simulink model "BEVModel"  (R2021a)
settings: Solver=ode4  StartTime=0  StopTime=tEnd  FixedStep=dt  RelTol=1e-3
values from neighbouring files (symbols this model uses):
  accessoryLoad = 600    [main.m]
  Af = 1.00    (= 1)    [main.m]
  batteryCapacity = 50    [main.m]
  batteryResistance = 0.0461    [main.m]
  C = 400    [main.m]
  Cd = 0.576    [main.m]
  Crr = 0.01    [main.m]
  cycleNum = 2    [main.m]
  EffTableEff = [.75 .85 .89 .95 .96 .97 .98 .99 .99]    [main.m]
  EffTableSpeed = [0 5 10 15 25 35 45 55 65]    [main.m]
  g = 9.81    [main.m]
  GRd = 9.843    [main.m]
  k_J2gal = 1/3600000/32.3    (= 8.59993120055e-09)    [main.m]
  k_kWh2J = 3.6*10^6    (= 3600000)    [main.m]
  k_m2mi = 0.000621371    [main.m]
  k_rps2rpm = 60/(2*pi)    (= 9.54929658551)    [main.m]
  k_s2h = 1/3600    (= 0.000277777777778)    [main.m]
  k_W2kW = 1/1000    (= 0.001)    [main.m]
  kc = 0.513    [main.m]
  Kd = 0    [main.m]
  Ki = 0.1    [main.m]
  ki = 0.0773    [main.m]
  Kp = 200    [main.m]
  kw = 0.0000064    (= 6.4e-06)    [main.m]
  m = 1965    [main.m]
  motorMaxPower = 310000    [main.m]
  motorMaxSpeed = 18000    [main.m]
  motorMaxTorque = 600    [main.m]
  openCircuitVoltage = 420    [main.m]
  pBrakeMax = 4*TbrakeMax / (mu_k*pi()* cylinderBore^2 *meanPadRadius*numPads)    [main.m]
  r = 0.290    (= 0.29)    [main.m]
  rho = 1.20    (= 1.2)    [main.m]
  SOCi = 90    [main.m]
  theta = 0    [main.m]
  v0 = 0    [main.m]
  x0 = 0    [main.m]
libraries: autolibshared x6, fl_lib x5, nesl_utility x5, sdl_lib x1
settings Model: Creator=Chris  LastModifiedBy=jordan
settings SolverCC: AlgebraicLoopSolver=TrustRegion
settings DebuggingCC: SFMachineParentedDataDiag=warning

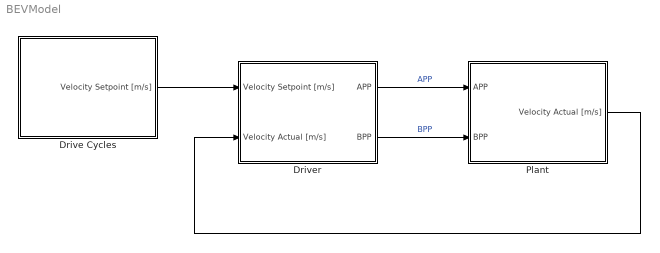
== system BEVModel ==
  Drive Cycles : Subsystem
  Driver : Subsystem
  Plant : Subsystem
  wires:
  Drive Cycles/1(Velocity Setpoint [m/s]) -> Driver/1(Velocity Setpoint [m/s])
  Driver/1(APP) -> Plant/1(APP)  "APP"
  Driver/2(BPP) -> Plant/2(BPP)  "BPP"
  Plant/1(Velocity Actual [m/s]) -> Driver/2(Velocity Actual [m/s])

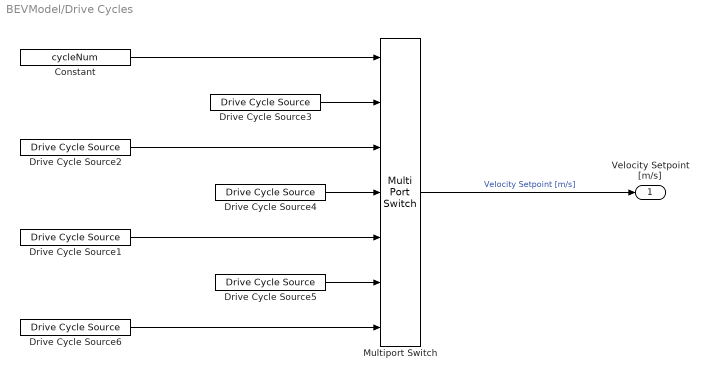
== system BEVModel/Drive Cycles ==
  Constant : Constant  Value=cycleNum
  Drive Cycle Source1 : autolibshared/Drive Cycle Source  cycleVar=HWFET  wsVar=driveCycle  fileVar=cycleFTP75.mat  tfinal="765  seconds"  cycleRepeat=off  outAccPort=off  outGearPort=off  gearList=No gear data  t_wot1=5  xdot_woto=0  xdot_wot1=30  t_wot2=20  xdot_wot2=0  t_wotend=30  srcUnit=m/s  outUnit=m/s  srcAccUnit=m/s/s  outAccUnit=m/s^2  dt=0  aMode=1  faultOption=off  velBnd=2  velBndUnit=mph  inUnit=m/s  timeBnd=1  failOption=off  stopSim=off  maxFaultCnt=10  maxFaultTime=2  maxTotFaultTime=15  traceOption=off  dtTrace=1  traceWindow=10  lastDCname=HWFET  lastOutUnit=mph  lastDT=0  lastTB=1  lastSB=2  forceCalcBound=off
      settings: SourceProductBaseCode=PW,DR,MT,UV,VE
  Drive Cycle Source2 : autolibshared/Drive Cycle Source  cycleVar=US06  wsVar=driveCycle  fileVar=cycleFTP75.mat  tfinal="600  seconds, Cyclic"  cycleRepeat=on  outAccPort=off  outGearPort=off  gearList=No gear data  t_wot1=5  xdot_woto=0  xdot_wot1=30  t_wot2=20  xdot_wot2=0  t_wotend=30  srcUnit=m/s  outUnit=m/s  srcAccUnit=m/s/s  outAccUnit=m/s^2  dt=0  aMode=1  faultOption=off  velBnd=2  velBndUnit=mph  inUnit=m/s  timeBnd=1  failOption=off  stopSim=off  maxFaultCnt=10  maxFaultTime=2  maxTotFaultTime=15  traceOption=off  dtTrace=1  traceWindow=10  lastDCname=US06  lastOutUnit=mph  lastDT=0  lastTB=1  lastSB=2  forceCalcBound=off
      settings: SourceProductBaseCode=PW,DR,MT,UV,VE
  Drive Cycle Source3 : autolibshared/Drive Cycle Source  cycleVar=Wide Open Throttle (WOT)  wsVar=driveCycle  fileVar=cycleFTP75.mat  tfinal="15  seconds, Cyclic"  cycleRepeat=on  outAccPort=off  outGearPort=off  gearList=No gear data  t_wot1=1  xdot_woto=0  xdot_wot1=vRef  t_wot2=tBrake  xdot_wot2=0  t_wotend=tEndWOT  srcUnit=m/s  outUnit=m/s  srcAccUnit=m/s/s  outAccUnit=m/s^2  dt=0  aMode=1  faultOption=off  velBnd=2  velBndUnit=mph  inUnit=m/s  timeBnd=1  failOption=off  stopSim=off  maxFaultCnt=10  maxFaultTime=2  maxTotFaultTime=15  traceOption=off  dtTrace=1  traceWindow=10  lastDCname=Custom Data Set  lastOutUnit=mph  lastDT=0  lastTB=1  lastSB=2  forceCalcBound=off
      settings: SourceProductBaseCode=PW,DR,MT,UV,VE
  Drive Cycle Source4 : autolibshared/Drive Cycle Source  cycleVar=UDDS  wsVar=driveCycle  fileVar=cycleFTP75.mat  tfinal="1369  seconds, Cyclic"  cycleRepeat=on  outAccPort=off  outGearPort=off  gearList=No gear data  t_wot1=1  xdot_woto=0  xdot_wot1=30  t_wot2=tBrake  xdot_wot2=0  t_wotend=tWOTEnd  srcUnit=m/s  outUnit=m/s  srcAccUnit=m/s/s  outAccUnit=m/s^2  dt=0  aMode=1  faultOption=off  velBnd=2  velBndUnit=mph  inUnit=m/s  timeBnd=1  failOption=off  stopSim=off  maxFaultCnt=10  maxFaultTime=2  maxTotFaultTime=15  traceOption=off  dtTrace=1  traceWindow=10  lastDCname=UDDS  lastOutUnit=mph  lastDT=0  lastTB=1  lastSB=2  forceCalcBound=off
      settings: SourceProductBaseCode=PW,DR,MT,UV,VE
  Drive Cycle Source5 : autolibshared/Drive Cycle Source  cycleVar=FTP75  wsVar=driveCycle  fileVar=cycleFTP75.mat  tfinal="2474  seconds"  cycleRepeat=off  outAccPort=off  outGearPort=off  gearList=No gear data  t_wot1=5  xdot_woto=0  xdot_wot1=30  t_wot2=20  xdot_wot2=0  t_wotend=30  srcUnit=m/s  outUnit=m/s  srcAccUnit=m/s/s  outAccUnit=m/s^2  dt=0  aMode=1  faultOption=off  velBnd=2  velBndUnit=mph  inUnit=m/s  timeBnd=1  failOption=off  stopSim=off  maxFaultCnt=10  maxFaultTime=2  maxTotFaultTime=15  traceOption=off  dtTrace=1  traceWindow=10  lastDCname=FTP75  lastOutUnit=mph  lastDT=0  lastTB=1  lastSB=2  forceCalcBound=off
      settings: SourceProductBaseCode=PW,DR,MT,UV,VE
  Drive Cycle Source6 : autolibshared/Drive Cycle Source  cycleVar=Wide Open Throttle (WOT)  wsVar=driveCycle  fileVar=cycleFTP75.mat  tfinal="15  seconds, Cyclic"  cycleRepeat=on  outAccPort=off  outGearPort=off  gearList=No gear data  t_wot1=1  xdot_woto=0  xdot_wot1=vRef  t_wot2=tBrake2  xdot_wot2=-50  t_wotend=tEndWOT2  srcUnit=mph  outUnit=m/s  srcAccUnit=m/s/s  outAccUnit=m/s^2  dt=0  aMode=1  faultOption=off  velBnd=2  velBndUnit=mph  inUnit=m/s  timeBnd=1  failOption=off  stopSim=off  maxFaultCnt=10  maxFaultTime=2  maxTotFaultTime=15  traceOption=off  dtTrace=1  traceWindow=10  lastDCname=Custom Data Set  lastOutUnit=mph  lastDT=0  lastTB=1  lastSB=2  forceCalcBound=off
      settings: SourceProductBaseCode=PW,DR,MT,UV,VE
  Multiport Switch : MultiPortSwitch  Inputs=6
  Velocity Setpoint [m/s] : Outport
  wires:
  Drive Cycle Source6/1 -> Multiport Switch/7
  Drive Cycle Source5/1 -> Multiport Switch/6
  Drive Cycle Source4/1 -> Multiport Switch/4
  Drive Cycle Source1/1 -> Multiport Switch/5
  Drive Cycle Source3/1 -> Multiport Switch/2
  Drive Cycle Source2/1 -> Multiport Switch/3
  Constant/1 -> Multiport Switch/1
  Multiport Switch/1 -> Velocity Setpoint [m/s]/1  "Velocity Setpoint [m/s]"

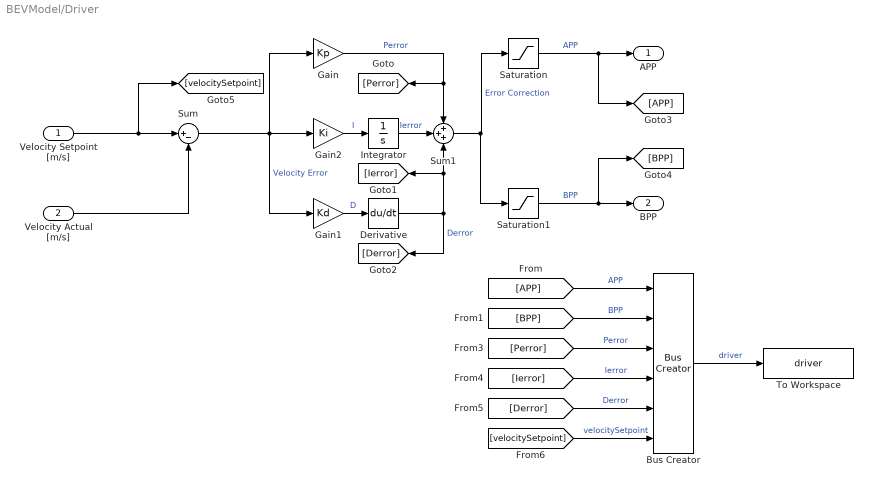
== system BEVModel/Driver ==
  Velocity Setpoint [m/s] : Inport
  Velocity Actual [m/s] : Inport  Port=2
  Bus Creator : BusCreator  Inputs=6
  Derivative : Derivative
  Gain : Gain  Gain=Kp
  Gain1 : Gain  Gain=Kd
  Gain2 : Gain  Gain=Ki
  Integrator : Integrator
  Saturation : Saturate  UpperLimit=100  LowerLimit=0
  Saturation1 : Saturate  UpperLimit=0  LowerLimit=-100
  Sum : Sum  Inputs=|+-
  Sum1 : Sum  Inputs=+++
  To Workspace : ToWorkspace  VariableName=driver  SaveFormat=Timeseries  SampleTime=-1
  APP : Outport
  BPP : Outport  Port=2
  wires:
  Gain/1 -> [Perror], Sum1/1  "Perror"
  Integrator/1 -> Sum1/2  "Ierror"
  Derivative/1 -> [Derror], [Ierror], Sum1/3  "Derror"
  Sum1/1 -> Saturation1/1, Saturation/1  "Error Correction"
  Sum/1 -> Gain2/1, Gain1/1, Gain/1  "Velocity Error"
  Velocity Setpoint [m/s]/1 -> [velocitySetpoint], Sum/1
  Velocity Actual [m/s]/1 -> Sum/2
  Saturation1/1 -> [BPP], BPP/1  "BPP"
  Saturation/1 -> [APP], APP/1  "APP"
  Gain2/1 -> Integrator/1  "I"
  Gain1/1 -> Derivative/1  "D"
  Bus Creator/1 -> To Workspace/1  "driver"
  [APP] -> Bus Creator/1  "APP"
  [BPP] -> Bus Creator/2  "BPP"
  [Perror] -> Bus Creator/3  "Perror"
  [Ierror] -> Bus Creator/4  "Ierror"
  [Derror] -> Bus Creator/5  "Derror"
  [velocitySetpoint] -> Bus Creator/6  "velocitySetpoint"

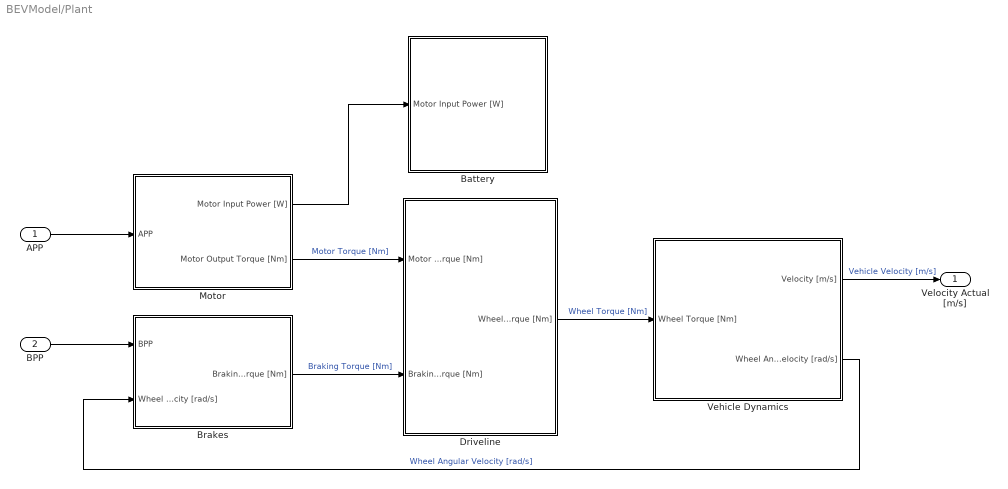
== system BEVModel/Plant ==
  APP : Inport
  BPP : Inport  Port=2
  Battery : Subsystem
  Brakes : Subsystem
  Driveline : Subsystem
  Motor : Subsystem
  Vehicle Dynamics : Subsystem
  Velocity Actual [m/s] : Outport
  wires:
  BPP/1 -> Brakes/1(BPP)
  Vehicle Dynamics/1(Velocity [m/s]) -> Velocity Actual [m/s]/1  "Vehicle Velocity [m/s]"
  Driveline/1(Wheel Torque [Nm]) -> Vehicle Dynamics/1(Wheel Torque [Nm])  "Wheel Torque [Nm]"
  Vehicle Dynamics/2(Wheel Angular Velocity [rad/s]) -> Brakes/2(Wheel Angular Velocity [rad/s])  "Wheel Angular Velocity [rad/s]"
  APP/1 -> Motor/1(APP)
  Motor/2(Motor Output Torque [Nm]) -> Driveline/1(Motor Torque [Nm])  "Motor Torque [Nm]"
  Motor/1(Motor Input Power [W]) -> Battery/1(Motor Input Power [W])
  Brakes/1(Braking Torque [Nm]) -> Driveline/2(Braking Torque [Nm])  "Braking Torque [Nm]"

== system BEVModel/Plant/Battery ==
  Motor Input Power [W] : Inport
  Current Calculation : Subsystem
  Energy Calculations and Data Management : Subsystem
  wires:
  Motor Input Power [W]/1 -> Current Calculation/1(Power to Motor [W])

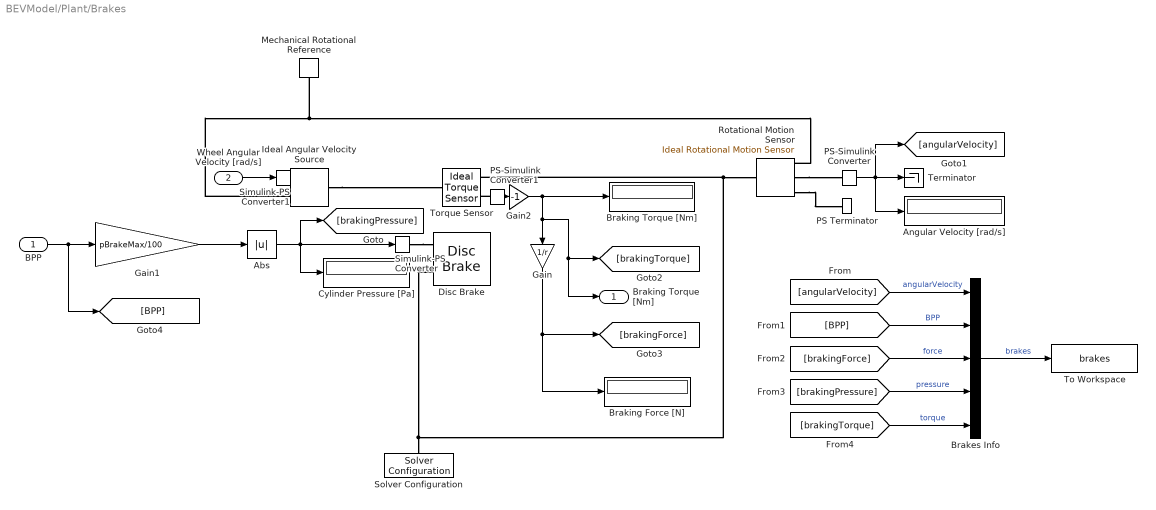
== system BEVModel/Plant/Brakes ==
  BPP : Inport
  Wheel Angular Velocity [rad/s] : Inport  Port=2
  Abs : Abs
  Angular Velocity [rad/s] : Display
  Brakes Info : BusCreator  Inputs=5
  Braking Force [N] : Display
  Braking Torque [Nm] : Display
  Cylinder Pressure [Pa] : Display
  Disc Brake : sdl_lib/Brakes & Detents/Rotational/Disc Brake  r_mean=meanPadRadius m  bore=cylinderBore m  n_pads=numPads  thermal_port=simscape.enum.thermaleffects.omit  mu_static=mu_s  mu_coulomb=mu_k  temperature_TLU=[280, 300, 320] K  mu_static_TLU=[.9, .8, .7]  mu_coulomb_TLU=[.8, .7, .6]  thermal_mass=50 kJ/K  brkwy_vel=omegaBreakAway rad/s  visc_coef=mu_v N*m/(rad/s)  enable_faults=simscape.enum.onoff.off  faulted_pressure=0 bar  external_fault=simscape.enum.onoff.off  temporal_fault=simscape.enum.onoff.off  fault_time=5 s  report_fault=simscape.enum.assert.action.none  temperature_specify=off  temperature_priority=High  temperature=300 K  temperature_nominal_specify=off  temperature_nominal_unit=K  temperature_nominal_value=1
      settings: SourceProductBaseCode=LD
  Gain : Gain  Gain=1/r
  Gain1 : Gain  Gain=pBrakeMax/100
  Gain2 : Gain  Gain=-1
  Ideal Angular Velocity Source : fl_lib/Mechanical/Mechanical Sources/Ideal Angular Velocity Source
  Mechanical Rotational Reference : fl_lib/Mechanical/Rotational Elements/Mechanical Rotational Reference
  PS Terminator : fl_lib/Physical Signals/Sinks/PS Terminator
  PS-Simulink Converter : nesl_utility/PS-Simulink Converter  PhysicalDomain=network_engine_domain  SubClassName=ps_output  LeftPortType=input  RightPortType=output  PseudoPeriodic=off  Frequencies=[]  Unit=inherit  AffineConversion=off
      settings: SourceProductBaseCode=PW,SS
  PS-Simulink Converter1 : nesl_utility/PS-Simulink Converter  PhysicalDomain=network_engine_domain  SubClassName=ps_output  LeftPortType=input  RightPortType=output  PseudoPeriodic=off  Frequencies=[]  Unit=inherit  AffineConversion=off
      settings: SourceProductBaseCode=PW,SS
  Rotational Motion Sensor : fl_lib/Mechanical/Mechanical Sensors/Ideal Rotational Motion Sensor  wrap_angle=simscape.enum.onoff.off  offset=0 rad
  Simulink-PS Converter : nesl_utility/Simulink-PS Converter  PhysicalDomain=network_engine_domain  SubClassName=ps_input  LeftPortType=input  RightPortType=output  PseudoPeriodic=off  Frequencies=[]  NoiseDistribution=none  NoiseParameters=[]  Unit=Pa  AffineConversion=off  FilteringAndDerivatives=provide  SimscapeFilterOrder=1  InputFilterTimeConstant=0.001  UdotUserProvided=0
      settings: SourceProductBaseCode=PW,SS
  Simulink-PS Converter1 : nesl_utility/Simulink-PS Converter  PhysicalDomain=network_engine_domain  SubClassName=ps_input  LeftPortType=input  RightPortType=output  PseudoPeriodic=off  Frequencies=[]  NoiseDistribution=none  NoiseParameters=[]  Unit=rad/s  AffineConversion=off  FilteringAndDerivatives=provide  SimscapeFilterOrder=1  InputFilterTimeConstant=0.001  UdotUserProvided=0
      settings: SourceProductBaseCode=PW,SS
  Solver Configuration : nesl_utility/Solver Configuration  PhysicalDomain=network_engine_domain  SubClassName=solver  LeftPortType=input  RightPortType=generic  Tones=[]  Harmonics=[]  SimulateNoise=off  Profile=off  UseLocalSampling=off  EnableSwitchedLinearOptims=on  FrequencyDomain=off  UseCCode=off  RelTol=0.001  AbsTol=1e-06  MinStep=1e-09  ToWorkspace=off  RevertToSquareIcSolve=off  NumHomotopyIterations=100  PhasorMode=off  PhasorModeNumHarmonics=1  DoDC=on  ResidualTolerance=1e-09  UseLocalSolver=on  LocalSolverChoice=NE_BACKWARD_EULER_ADVANCER  LocalSolverSampleTime=0.01  DoFixedCost=on  MaxNonlinIter=3  MaxModeIter=2  ComputeImpulses=off  ImpulseIterations=2  LinearAlgebra=auto  EquationFormulation=NE_TIME_EF  DelaysMemoryBudget=1024  AutomaticFiltering=on  FilteringTimeConstant=0.001  PartitionStorageMethod=AS_NEEDED  PartitionMemoryBudget=1024  PartitionMethod=ROBUST
      settings: SourceProductBaseCode=PW,SS
  Terminator : Terminator
  To Workspace : ToWorkspace  VariableName=brakes  SaveFormat=Timeseries  SampleTime=-1
  Torque Sensor : fl_lib/Mechanical/Mechanical Sensors/Ideal Torque Sensor
  Braking Torque [Nm] : Outport
  wires:
  Gain/1 -> Braking Force [N]/1, [brakingForce]
  Gain2/1 -> Braking Torque [Nm]/1, [brakingTorque], Braking Torque [Nm]/1, Gain/1
  PS-Simulink Converter/1 -> [angularVelocity], Angular Velocity [rad/s]/1, Terminator/1
  Abs/1 -> [brakingPressure], Cylinder Pressure [Pa]/1, Simulink-PS Converter/1
  Gain1/1 -> Abs/1
  BPP/1 -> [BPP], Gain1/1
  [angularVelocity] -> Brakes Info/1  "angularVelocity"
  [BPP] -> Brakes Info/2  "BPP"
  [brakingForce] -> Brakes Info/3  "force"
  [brakingPressure] -> Brakes Info/4  "pressure"
  [brakingTorque] -> Brakes Info/5  "torque"
  Brakes Info/1 -> To Workspace/1  "brakes"
  PS-Simulink Converter1/1 -> Gain2/1
  Wheel Angular Velocity [rad/s]/1 -> Simulink-PS Converter1/1
  connections:
  Simulink-PS Converter1/RConn1 -- Ideal Angular Velocity Source/RConn1
  Rotational Motion Sensor/RConn2 -- PS-Simulink Converter/LConn1
  Torque Sensor/RConn1 -- Rotational Motion Sensor/LConn1 -- Disc Brake/LConn2 -- Solver Configuration/RConn1
  Ideal Angular Velocity Source/RConn2 -- Rotational Motion Sensor/RConn1 -- Mechanical Rotational Reference/LConn1
  Ideal Angular Velocity Source/LConn1 -- Torque Sensor/LConn1
  Rotational Motion Sensor/RConn3 -- PS Terminator/LConn1
  Simulink-PS Converter/RConn1 -- Disc Brake/LConn1
  PS-Simulink Converter1/LConn1 -- Torque Sensor/RConn2

== system BEVModel/Plant/Driveline ==
  Motor Torque [Nm] : Inport
  Braking Torque [Nm] : Inport  Port=2
  Efficiency Look-up Table : Lookup_n-D  NumberOfTableDimensions=1  BreakpointsForDimension1=EffTableSpeed  Table=EffTableEff  InternalRulePriority=Speed  RndMeth=Simplest  InputSameDT=on
  Gain1 : Gain  Gain=GRd
  Product1 : Product
  Sum1 : Sum
  Wheel Torque [Nm] : Outport
  wires:
  Motor Torque [Nm]/1 -> Gain1/1
  Gain1/1 -> Product1/2  "Positive Torque [N-m]"
  Braking Torque [Nm]/1 -> Sum1/2  "Braking Torque [N-m]"
  Sum1/1 -> Wheel Torque [Nm]/1
  [velocityActual] -> Efficiency Look-up Table/1  "Velocity Actual [m/s]"
  Efficiency Look-up Table/1 -> Product1/1  "Driveline Efficiency"
  Product1/1 -> Sum1/1

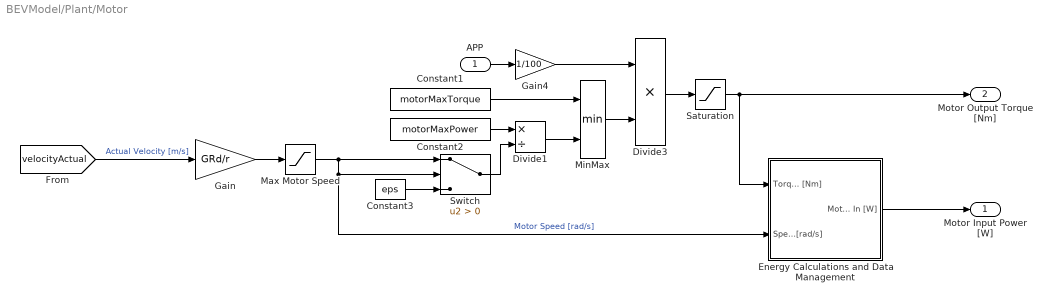
== system BEVModel/Plant/Motor ==
  APP : Inport
  Constant1 : Constant  Value=motorMaxTorque
  Constant2 : Constant  Value=motorMaxPower
  Constant3 : Constant  Value=eps
  Divide1 : Product  Inputs=*/
  Divide3 : Product  Inputs=**
  Energy Calculations and Data Management : Subsystem
  Gain : Gain  Gain=GRd/r
  Gain4 : Gain  Gain=1/100
  Max Motor Speed : Saturate  UpperLimit=motorMaxSpeed/k_rps2rpm  LowerLimit=0
  MinMax : MinMax  Inputs=2
  Saturation : Saturate  UpperLimit=motorMaxTorque  LowerLimit=0
  Switch : Switch  Criteria=u2 > Threshold
  Motor Input Power [W] : Outport
  Motor Output Torque [Nm] : Outport  Port=2
  wires:
  Gain/1 -> Max Motor Speed/1
  [velocityActual] -> Gain/1  "Actual Velocity [m/s]"
  APP/1 -> Gain4/1
  Constant1/1 -> MinMax/1
  Constant3/1 -> Switch/3
  Divide1/1 -> MinMax/2
  Divide3/1 -> Saturation/1
  Saturation/1 -> Motor Output Torque [Nm]/1, Energy Calculations and Data Management/1(Torque [Nm])
  Max Motor Speed/1 -> Energy Calculations and Data Management/2(Speed [rad/s]), Switch/2, Switch/1  "Motor Speed [rad/s]"
  Switch/1 -> Divide1/2
  Constant2/1 -> Divide1/1
  Gain4/1 -> Divide3/1
  MinMax/1 -> Divide3/2
  Energy Calculations and Data Management/1(Motor Power In [W]) -> Motor Input Power [W]/1

== system BEVModel/Plant/Vehicle Dynamics ==
  Wheel Torque [Nm] : Inport
  Data Management : Subsystem
  Dynamics Calculations : Subsystem
  Energy Calculations : Subsystem
  Velocity [m/s] : Outport
  Wheel Angular Velocity [rad/s] : Outport  Port=2
  wires:
  Wheel Torque [Nm]/1 -> Dynamics Calculations/1(Wheel Torque [Nm])  "Wheel Torque [Nm]"
  Dynamics Calculations/1(Tractive Force [N]) -> Energy Calculations/1(Tractive Force [N])
  Dynamics Calculations/2(Velocity [m/s]) -> Energy Calculations/2(Velocity [m/s]), Velocity [m/s]/1
  Dynamics Calculations/3(Rolling Resistance [N]) -> Energy Calculations/3(Rolling Resistance [N])
  Dynamics Calculations/4(Grade Force [N]) -> Energy Calculations/4(Grade Force [N])
  Dynamics Calculations/5(Drag Force [N]) -> Energy Calculations/5(Drag Force [N])
  Dynamics Calculations/6(Angular Velocity [rad/s]) -> Wheel Angular Velocity [rad/s]/1, Energy Calculations/6(Angular Velocity [rad/s])

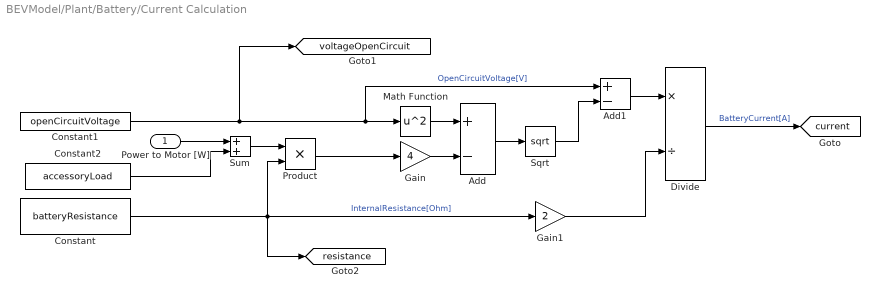
== system BEVModel/Plant/Battery/Current Calculation ==
  Power to Motor [W] : Inport
  Add : Sum  Inputs=+-
  Add1 : Sum  Inputs=+-
  Constant : Constant  Value=batteryResistance
  Constant1 : Constant  Value=openCircuitVoltage  SampleTime=-1
  Constant2 : Constant  Value=accessoryLoad
  Divide : Product  Inputs=*/
  Gain : Gain  Gain=4
  Gain1 : Gain  Gain=2
  Math Function : Math  Operator=square  SignedPower=on  SaturateOnIntegerOverflow=on
  Product : Product  RndMeth=Zero
  Sqrt : Sqrt  SaturateOnIntegerOverflow=on
  Sum : Sum
  tag scope: current=global, resistance=global, voltageOpenCircuit=global
  wires:
  Math Function/1 -> Add/1
  Gain/1 -> Add/2
  Add/1 -> Sqrt/1
  Constant/1 -> Product/2, Gain1/1, [resistance]  "InternalResistance[Ohm]"
  Sqrt/1 -> Add1/2
  Divide/1 -> [current]  "BatteryCurrent[A]"
  Power to Motor [W]/1 -> Sum/1
  Product/1 -> Gain/1
  Add1/1 -> Divide/1
  Gain1/1 -> Divide/2
  Constant1/1 -> [voltageOpenCircuit], Add1/1, Math Function/1  "OpenCircuitVoltage[V]"
  Constant2/1 -> Sum/2
  Sum/1 -> Product/1

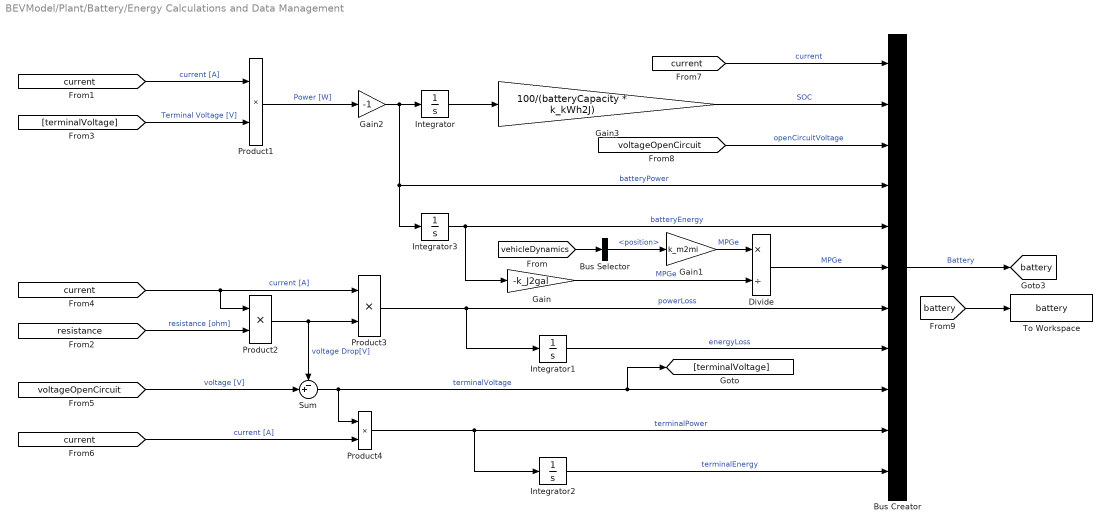
== system BEVModel/Plant/Battery/Energy Calculations and Data Management ==
  Bus Creator : BusCreator  Inputs=11
  Bus Selector : BusSelector  OutputSignals=position
  Divide : Product  Inputs=*/
  Gain : Gain  Gain=-k_J2gal
  Gain1 : Gain  Gain=k_m2mi
  Gain2 : Gain  Gain=-1
  Gain3 : Gain  Gain=100/(batteryCapacity * k_kWh2J)
  Integrator : Integrator  InitialCondition=SOCi/100 * batteryCapacity * k_kWh2J
  Integrator1 : Integrator
  Integrator2 : Integrator
  Integrator3 : Integrator
  Product1 : Product
  Product2 : Product
  Product3 : Product
  Product4 : Product  Inputs=**
  Sum : Sum  Inputs=-+|
  To Workspace : ToWorkspace  VariableName=battery  SaveFormat=Timeseries  SampleTime=-1
  tag scope: battery=global
  wires:
  Integrator/1 -> Gain3/1
  [current] -> Product1/1  "current [A]"
  Gain3/1 -> Bus Creator/2  "SOC"
  Integrator1/1 -> Bus Creator/8  "energyLoss"
  [current] -> Product3/1, Product2/1  "current [A]"
  Gain2/1 -> Bus Creator/4, Integrator3/1, Integrator/1  "batteryPower"
  Product1/1 -> Gain2/1  "Power [W]"
  Product4/1 -> Integrator2/1, Bus Creator/10  "terminalPower"
  [resistance] -> Product2/2  "resistance [ohm]"
  Product2/1 -> Product3/2, Sum/1  "voltage Drop[V]"
  Bus Creator/1 -> [battery]  "Battery"
  Product3/1 -> Bus Creator/7, Integrator1/1  "powerLoss"
  [voltageOpenCircuit] -> Sum/2  "voltage [V]"
  Sum/1 -> [terminalVoltage], Bus Creator/9, Product4/1  "terminalVoltage"
  [current] -> Bus Creator/1  "current"
  [current] -> Product4/2  "current [A]"
  Integrator2/1 -> Bus Creator/11  "terminalEnergy"
  [voltageOpenCircuit] -> Bus Creator/3  "openCircuitVoltage"
  Integrator3/1 -> Bus Creator/5, Gain/1  "batteryEnergy"
  Divide/1 -> Bus Creator/6  "MPGe"
  [vehicleDynamics] -> Bus Selector/1
  Bus Selector/1 -> Gain1/1  "<position>"
  Gain1/1 -> Divide/1  "MPGe"
  Gain/1 -> Divide/2  "MPGe"
  [battery] -> To Workspace/1
  [terminalVoltage] -> Product1/2  "Terminal Voltage [V]"

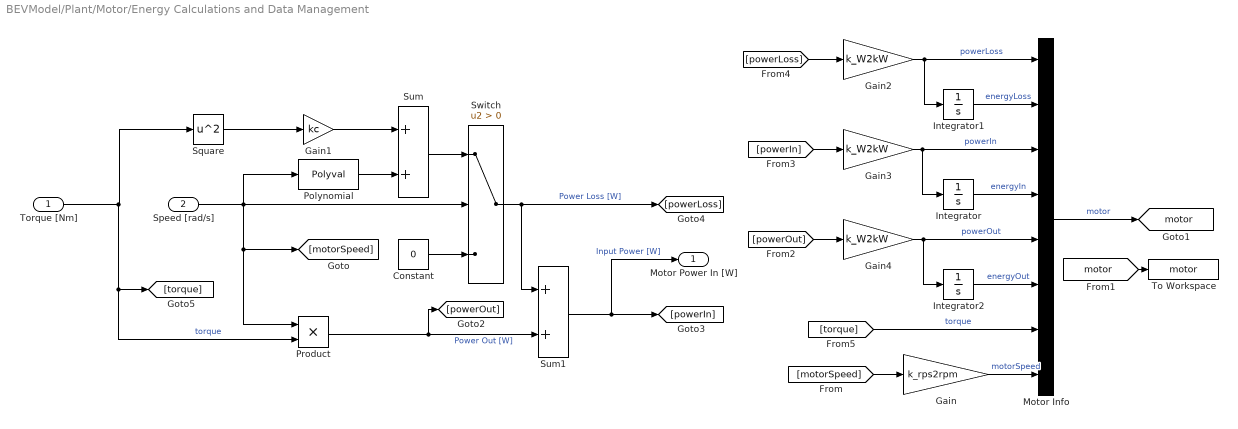
== system BEVModel/Plant/Motor/Energy Calculations and Data Management ==
  Torque [Nm] : Inport
  Speed [rad/s] : Inport  Port=2
  Constant : Constant  Value=0
  Gain : Gain  Gain=k_rps2rpm
  Gain1 : Gain  Gain=kc
  Gain2 : Gain  Gain=k_W2kW
  Gain3 : Gain  Gain=k_W2kW
  Gain4 : Gain  Gain=k_W2kW
  Integrator : Integrator
  Integrator1 : Integrator
  Integrator2 : Integrator
  Motor Info : BusCreator  Inputs=8
  Polynomial : Polyval  Coefs=[kw , 0 ki, C]
  Product : Product
  Square : Math  Operator=square  SaturateOnIntegerOverflow=on
  Sum : Sum
  Sum1 : Sum
  Switch : Switch  Criteria=u2 > Threshold
  To Workspace : ToWorkspace  VariableName=motor  SaveFormat=Timeseries  SampleTime=-1
  Motor Power In [W] : Outport
  tag scope: motor=global
  wires:
  Motor Info/1 -> [motor]  "motor"
  Product/1 -> [powerOut], Sum1/2  "Power Out [W]"
  Speed [rad/s]/1 -> Polynomial/1, Product/1, [motorSpeed], Switch/2
  Constant/1 -> Switch/3
  Polynomial/1 -> Sum/2
  Sum/1 -> Switch/1
  Gain1/1 -> Sum/1
  Switch/1 -> Sum1/1, [powerLoss]  "Power Loss [W]"
  Sum1/1 -> Motor Power In [W]/1, [powerIn]  "Input Power [W]"
  Torque [Nm]/1 -> Square/1, Product/2, [torque]  "torque"
  Square/1 -> Gain1/1
  Integrator/1 -> Motor Info/4  "energyIn"
  Integrator2/1 -> Motor Info/6  "energyOut"
  Integrator1/1 -> Motor Info/2  "energyLoss"
  [motorSpeed] -> Gain/1
  Gain/1 -> Motor Info/8  "motorSpeed"
  [motor] -> To Workspace/1
  Gain4/1 -> Integrator2/1, Motor Info/5  "powerOut"
  Gain3/1 -> Motor Info/3, Integrator/1  "powerIn"
  Gain2/1 -> Motor Info/1, Integrator1/1  "powerLoss"
  [torque] -> Motor Info/7  "torque"
  [powerLoss] -> Gain2/1
  [powerIn] -> Gain3/1
  [powerOut] -> Gain4/1

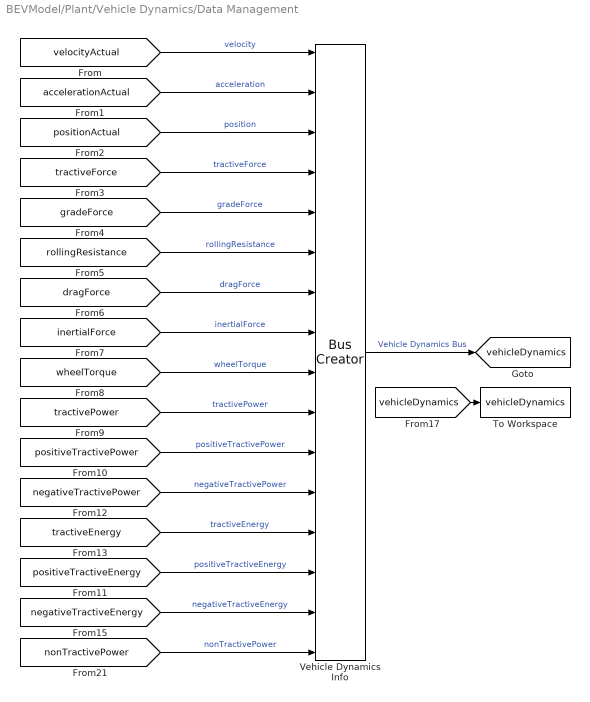
== system BEVModel/Plant/Vehicle Dynamics/Data Management ==
  To Workspace : ToWorkspace  VariableName=vehicleDynamics  SaveFormat=Timeseries  SampleTime=-1
  Vehicle Dynamics Info : BusCreator  Inputs=16
  tag scope: vehicleDynamics=global
  wires:
  [velocityActual] -> Vehicle Dynamics Info/1  "velocity"
  [wheelTorque] -> Vehicle Dynamics Info/9  "wheelTorque"
  [tractiveForce] -> Vehicle Dynamics Info/4  "tractiveForce"
  [negativeTractivePower] -> Vehicle Dynamics Info/12  "negativeTractivePower"
  [accelerationActual] -> Vehicle Dynamics Info/2  "acceleration"
  [vehicleDynamics] -> To Workspace/1
  [gradeForce] -> Vehicle Dynamics Info/5  "gradeForce"
  [positiveTractivePower] -> Vehicle Dynamics Info/11  "positiveTractivePower"
  [positiveTractiveEnergy] -> Vehicle Dynamics Info/14  "positiveTractiveEnergy"
  [rollingResistance] -> Vehicle Dynamics Info/6  "rollingResistance"
  [inertialForce] -> Vehicle Dynamics Info/8  "inertialForce"
  [positionActual] -> Vehicle Dynamics Info/3  "position"
  [tractivePower] -> Vehicle Dynamics Info/10  "tractivePower"
  [negativeTractiveEnergy] -> Vehicle Dynamics Info/15  "negativeTractiveEnergy"
  [tractiveEnergy] -> Vehicle Dynamics Info/13  "tractiveEnergy"
  [dragForce] -> Vehicle Dynamics Info/7  "dragForce"
  [nonTractivePower] -> Vehicle Dynamics Info/16  "nonTractivePower"
  Vehicle Dynamics Info/1 -> [vehicleDynamics]  "Vehicle Dynamics Bus"

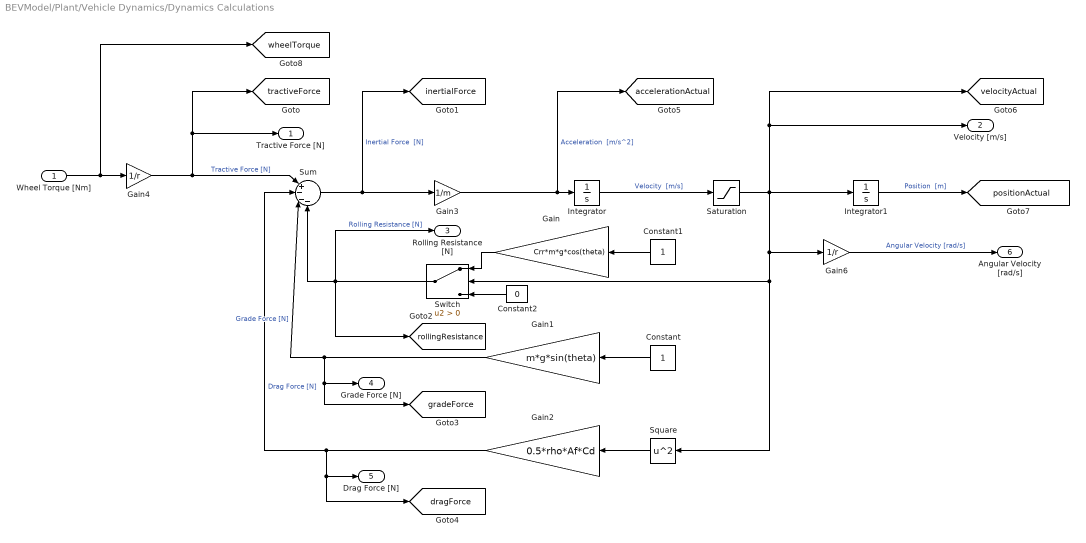
== system BEVModel/Plant/Vehicle Dynamics/Dynamics Calculations ==
  Wheel Torque [Nm] : Inport
  Constant : Constant
  Constant1 : Constant
  Constant2 : Constant  Value=0
  Gain : Gain  Gain=Crr*m*g*cos(theta)
  Gain1 : Gain  Gain=m*g*sin(theta)
  Gain2 : Gain  Gain=0.5*rho*Af*Cd
  Gain3 : Gain  Gain=1/m
  Gain4 : Gain  Gain=1/r
  Gain6 : Gain  Gain=1/r
  Integrator : Integrator  InitialCondition=v0
  Integrator1 : Integrator  InitialCondition=x0
  Saturation : Saturate  UpperLimit=inf  LowerLimit=0  LinearizeAsGain=off
  Square : Math  Operator=square  SaturateOnIntegerOverflow=on
  Sum : Sum  Inputs=|+---
  Switch : Switch  Criteria=u2 > Threshold
  Tractive Force [N] : Outport
  Velocity [m/s] : Outport  Port=2
  Rolling Resistance [N] : Outport  Port=3
  Grade Force [N] : Outport  Port=4
  Drag Force [N] : Outport  Port=5
  Angular Velocity [rad/s] : Outport  Port=6
  tag scope: accelerationActual=global, dragForce=global, gradeForce=global, inertialForce=global, positionActual=global, rollingResistance=global, tractiveForce=global, velocityActual=global, wheelTorque=global
  wires:
  Gain1/1 -> Grade Force [N]/1, [gradeForce], Sum/3  "Grade Force [N]"
  Gain4/1 -> Tractive Force [N]/1, [tractiveForce], Sum/1  "Tractive Force [N]"
  Constant/1 -> Gain1/1
  Switch/1 -> Sum/4, [rollingResistance], Rolling Resistance [N]/1  "Rolling Resistance [N]"
  Integrator/1 -> Saturation/1  "Velocity  [m/s]"
  Integrator1/1 -> [positionActual]  "Position  [m]"
  Sum/1 -> [inertialForce], Gain3/1  "Inertial Force  [N]"
  Constant1/1 -> Gain/1
  Gain3/1 -> [accelerationActual], Integrator/1  "Acceleration  [m/s^2]"
  Gain2/1 -> Drag Force [N]/1, [dragForce], Sum/2  "Drag Force [N]"
  Wheel Torque [Nm]/1 -> [wheelTorque], Gain4/1
  Square/1 -> Gain2/1
  Saturation/1 -> Gain6/1, Square/1, Switch/2, Velocity [m/s]/1, [velocityActual], Integrator1/1
  Gain/1 -> Switch/1
  Constant2/1 -> Switch/3
  Gain6/1 -> Angular Velocity [rad/s]/1  "Angular Velocity [rad/s]"

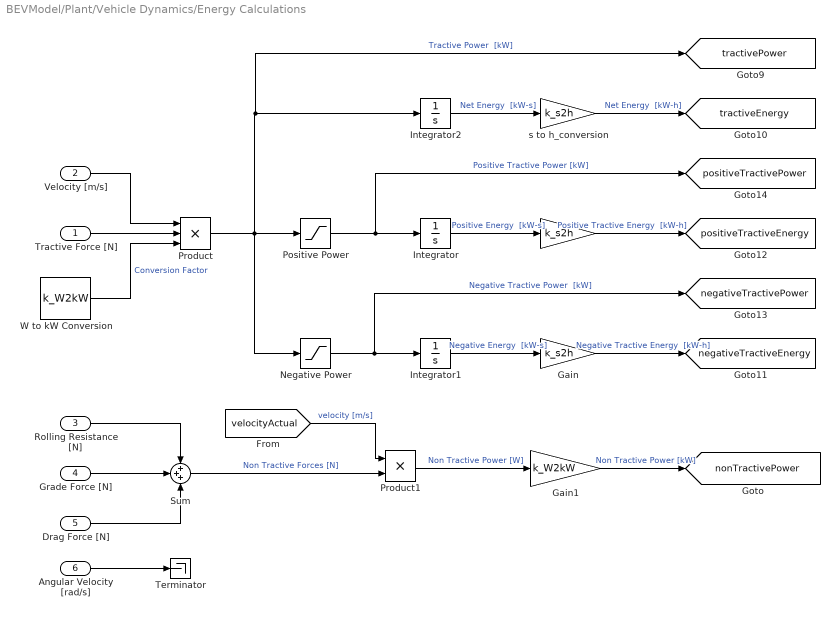
== system BEVModel/Plant/Vehicle Dynamics/Energy Calculations ==
  Tractive Force [N] : Inport
  Velocity [m/s] : Inport  Port=2
  Rolling Resistance [N] : Inport  Port=3
  Grade Force [N] : Inport  Port=4
  Drag Force [N] : Inport  Port=5
  Angular Velocity [rad/s] : Inport  Port=6
  " " : Gain  Gain=k_s2h
  Gain : Gain  Gain=k_s2h
  Gain1 : Gain  Gain=k_W2kW
  Integrator : Integrator
  Integrator1 : Integrator
  Integrator2 : Integrator
  Negative Power : Saturate  UpperLimit=0  LowerLimit=-inf
  Positive Power : Saturate  UpperLimit=inf  LowerLimit=0
  Product : Product  Inputs=3
  Product1 : Product
  Sum : Sum  Inputs=+++
  Terminator : Terminator
  W to kW Conversion : Constant  Value=k_W2kW
  s to h_conversion : Gain  Gain=k_s2h
  tag scope: negativeTractiveEnergy=global, negativeTractivePower=global, nonTractivePower=global, positiveTractiveEnergy=global, positiveTractivePower=global, tractiveEnergy=global, tractivePower=global
  wires:
  s to h_conversion/1 -> [tractiveEnergy]  "Net Energy  [kW-h]"
  " "/1 -> [positiveTractiveEnergy]  "Positive Tractive Energy  [kW-h]"
  Gain/1 -> [negativeTractiveEnergy]  "Negative Tractive Energy  [kW-h]"
  Integrator1/1 -> Gain/1  "Negative Energy  [kW-s]"
  Integrator/1 -> " "/1  "Positive Energy  [kW-s]"
  Negative Power/1 -> [negativeTractivePower], Integrator1/1  "Negative Tractive Power  [kW]"
  Integrator2/1 -> s to h_conversion/1  "Net Energy  [kW-s]"
  Positive Power/1 -> [positiveTractivePower], Integrator/1  "Positive Tractive Power [kW]"
  W to kW Conversion/1 -> Product/3  "Conversion Factor"
  Product/1 -> Negative Power/1, [tractivePower], Integrator2/1, Positive Power/1  "Tractive Power  [kW]"
  Velocity [m/s]/1 -> Product/1
  Tractive Force [N]/1 -> Product/2
  Drag Force [N]/1 -> Sum/3
  Grade Force [N]/1 -> Sum/2
  Rolling Resistance [N]/1 -> Sum/1
  Sum/1 -> Product1/2  "Non Tractive Forces [N]"
  [velocityActual] -> Product1/1  "velocity [m/s]"
  Product1/1 -> Gain1/1  "Non Tractive Power [W]"
  Gain1/1 -> [nonTractivePower]  "Non Tractive Power [kW]"
  Angular Velocity [rad/s]/1 -> Terminator/1
